simulink model "npc_controller"  (R2022a)
settings: Solver=FixedStepDiscrete  StartTime=0.0  StopTime=20  RelTol=1e-3  EnableMultiTasking=on
values from neighbouring files (symbols this model uses):
  Tsw = 1.5E-5    [param.sldd]
undefined symbols (not defined in the file or in its folder): CAN_O_INT, CANA_BASE, Down, GPTRIP1SEL, GPTRIP2SEL, GPTRIP3SEL, TZ1, TZ2, TZ3, Up
libraries: simulink x153, hdlsllib x90, c2802xlib x34, c2837xDlib x18, c280xlib x12, canmsglib x9, c2838xlib x8, idelinklib_common x3, c2806xlib x2, slpidlib x2, c28004xlib x2, c281xlib x2
(part 34 of 45)

== system npc_controller/CONTROL/CONTROL/false/CLA_CONTROL/CONTROL/vloop_pi_parallel ==
  note: okay til 0.1A load
  note: Parallel PI
  note: div10
  error : Inport
  Constant : Constant  Commented=on  Value=1.06066  OutDataTypeStr=single
  Constant1 : Constant  Commented=on  Value=0.00106066  OutDataTypeStr=single
  Constant10 : Constant  Commented=on  Value=0.000056066  OutDataTypeStr=single
  Constant11 : Constant  Value=-32*25.324  OutDataTypeStr=single
  Constant12 : Constant  Commented=on  Value=0  OutDataTypeStr=single
  Constant13 : Constant  Value=0.00056066  OutDataTypeStr=single
  Constant2 : Constant  Value=32*25.324  OutDataTypeStr=single
  Constant3 : Constant  Commented=on  Value=0.0056066  OutDataTypeStr=single
  Constant4 : Constant  OutDataTypeStr=single
  Constant5 : Constant  Value=0.56066  OutDataTypeStr=single
  Constant6 : Constant  Commented=on  Value=0.0056066  OutDataTypeStr=single
  Constant7 : Constant  Commented=on  Value=0.56066  OutDataTypeStr=single
  Constant8 : Constant  Commented=on  Value=0.00056066  OutDataTypeStr=single
  Constant9 : Constant  Commented=on  Value=0.056066  OutDataTypeStr=single
  Delay1 : Delay  DelayLength=1  InitialCondition=0  StateName=vbulk_pid1  StateMustResolveToSignalObject=on
  Product2 : Product  Inputs=3  OutDataTypeStr=single
  Product3 : Product  OutDataTypeStr=single
  Saturation Dynamic : simulink/Discontinuities/Saturation Dynamic  OutMin=[]  OutMax=[]  OutDataTypeStr=single  OutputDataTypeScalingMode=single  OutDataType=fixdt(1, 16)  OutScaling=2^-10  DoSatur=off
  Saturation Dynamic1 : simulink/Discontinuities/Saturation Dynamic  OutMin=[]  OutMax=[]  OutDataTypeStr=single  OutputDataTypeScalingMode=single  OutDataType=fixdt(1, 16)  OutScaling=2^-10  DoSatur=off
  Scope : Scope  NumInputPorts=4
  Sum : Sum  Inputs=|++  AccumDataTypeStr=single  OutDataTypeStr=single
  Sum3 : Sum  Inputs=|++  AccumDataTypeStr=single  OutDataTypeStr=single
  pi : Outport
  wires:
  [error] -> Scope/1  "error"
  [kP_term] -> Scope/2  "kP_term"
  [kI_term] -> Scope/3  "kI_term"
  [pi] -> Scope/4  "PI"
  [Ts] -> Product2/3
  Constant4/1 -> [Ts]
  [kp] -> Product3/2
  [integ_min] -> Saturation Dynamic/3
  Sum/1 -> Saturation Dynamic1/2
  [integ_min] -> Saturation Dynamic1/3
  [integ_max] -> Saturation Dynamic1/1
  Constant2/1 -> [integ_max]
  Constant11/1 -> [integ_min]
  Product2/1 -> Sum3/1
  Product3/1 -> Sum/1, [kP_term]
  [error] -> Product3/1
  Constant13/1 -> [ki]
  [integ_max] -> Saturation Dynamic/1
  [error] -> Product2/1
  error/1 -> [error]
  Saturation Dynamic/1 -> [kI_term], Sum/2, Delay1/1
  [ki] -> Product2/2
  Saturation Dynamic1/1 -> pi/1, [pi]
  Constant5/1 -> [kp]
  Sum3/1 -> Saturation Dynamic/2
  Delay1/1 -> Sum3/2

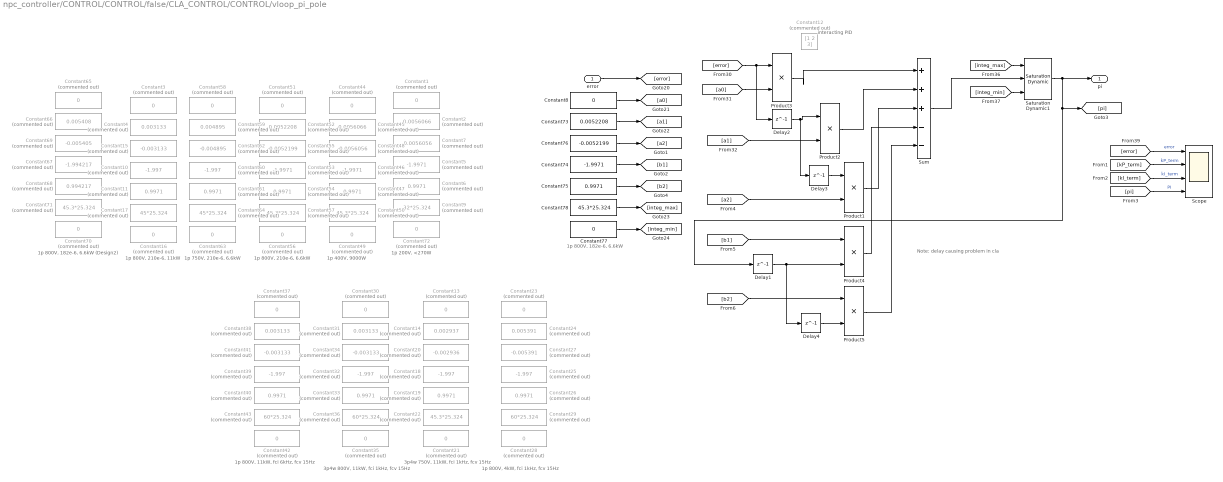
== system npc_controller/CONTROL/CONTROL/false/CLA_CONTROL/CONTROL/vloop_pi_pole ==
  note: interacting PID
  note: Note: delay causing problem in cla
  note: 1p 200V, <270W
  note: 3p4w 750V, 11kW, fci 1kHz, fcv 15Hz
  note: 1p 800V, 4kW, fci 1kHz, fcv 15Hz
  note: 3p4w 800V, 11kW, fci 1kHz, fcv 15Hz
  note: 1p 800V, 11kW, fci 6kHz, fcv 15Hz
  note: 1p 750V, 210e-6, 6.6kW
  note: 1p 800V, 210e-6, 6.6kW
  note: 1p 800V, 210e-6, 11kW
  note: 1p 800V, 182e-6, 6.6kW (Design2)
  note: 1p 400V, 9000W
  note: 1p 800V, 182e-6, 6.6kW
  error : Inport  OutDataTypeStr=single
  Constant{1,3,13,23,30,37,44,51,58,65} (10 alike) : Constant  Commented=on  Value=0  VectorParams1D=off  OutDataTypeStr=single
  Constant{10,18,25,32,39,60} (6 alike) : Constant  Commented=on  Value=-1.997  OutDataTypeStr=single
  Constant{6,11,19,26,33,40,47,54,61} (9 alike) : Constant  Commented=on  Value=0.9971  OutDataTypeStr=single
  Constant12 : Constant  Commented=on  Value=[1 2 3]  OutDataTypeStr=single
  Constant14 : Constant  Commented=on  Value=0.002937  OutDataTypeStr=single
  Constant15 : Constant  Commented=on  Value=-0.003133  OutDataTypeStr=single
  Constant{16,21,28,35,42,49,56,63,70,72} (10 alike) : Constant  Commented=on  Value=0  OutDataTypeStr=single
  Constant17 : Constant  Commented=on  Value=45*25.324  OutDataTypeStr=single
  Constant2 : Constant  Commented=on  Value=0.0056066  OutDataTypeStr=single
  Constant20 : Constant  Commented=on  Value=-0.002936  OutDataTypeStr=single
  Constant{22,50,57,71} (4 alike) : Constant  Commented=on  Value=45.3*25.324  OutDataTypeStr=single
  Constant24 : Constant  Commented=on  Value=0.005391  OutDataTypeStr=single
  Constant27 : Constant  Commented=on  Value=-0.005391  OutDataTypeStr=single
  Constant29 : Constant  Commented=on  Value=60*25.324  OutDataTypeStr=single
  Constant31 : Constant  Commented=on  Value=0.003133  OutDataTypeStr=single
  Constant34 : Constant  Commented=on  Value=-0.003133  OutDataTypeStr=single
  Constant36 : Constant  Commented=on  Value=60*25.324  OutDataTypeStr=single
  Constant38 : Constant  Commented=on  Value=0.003133  OutDataTypeStr=single
  Constant4 : Constant  Commented=on  Value=0.003133  OutDataTypeStr=single
  Constant41 : Constant  Commented=on  Value=-0.003133  OutDataTypeStr=single
  Constant43 : Constant  Commented=on  Value=60*25.324  OutDataTypeStr=single
  Constant45 : Constant  Commented=on  Value=0.0056066  OutDataTypeStr=single
  Constant46 : Constant  Commented=on  Value=-1.9971  OutDataTypeStr=single
  Constant48 : Constant  Commented=on  Value=-0.0056056  OutDataTypeStr=single
  Constant5 : Constant  Commented=on  Value=-1.9971  OutDataTypeStr=single
  Constant52 : Constant  Commented=on  Value=0.0052208  OutDataTypeStr=single
  Constant53 : Constant  Commented=on  Value=-1.9971  OutDataTypeStr=single
  Constant55 : Constant  Commented=on  Value=-0.0052199  OutDataTypeStr=single
  Constant59 : Constant  Commented=on  Value=0.004895  OutDataTypeStr=single
  Constant62 : Constant  Commented=on  Value=-0.004895  OutDataTypeStr=single
  Constant64 : Constant  Commented=on  Value=45*25.324  OutDataTypeStr=single
  Constant66 : Constant  Commented=on  Value=0.005408  OutDataTypeStr=single
  Constant67 : Constant  Commented=on  Value=-1.994217  OutDataTypeStr=single
  Constant68 : Constant  Commented=on  Value=0.994217  OutDataTypeStr=single
  Constant69 : Constant  Commented=on  Value=-0.005405  OutDataTypeStr=single
  Constant7 : Constant  Commented=on  Value=-0.0056056  OutDataTypeStr=single
  Constant73 : Constant  Value=0.0052208  OutDataTypeStr=single
  Constant74 : Constant  Value=-1.9971  OutDataTypeStr=single
  Constant75 : Constant  Value=0.9971  OutDataTypeStr=single
  Constant76 : Constant  Value=-0.0052199  OutDataTypeStr=single
  Constant77 : Constant  Value=0  OutDataTypeStr=single
  Constant78 : Constant  Value=45.3*25.324  OutDataTypeStr=single
  Constant8 : Constant  Value=0  VectorParams1D=off  OutDataTypeStr=single
  Constant9 : Constant  Commented=on  Value=32*25.324  OutDataTypeStr=single
  Delay1 : Delay  DelayLength=1  InitialCondition=0  StateName=vbulk_pid3  StateMustResolveToSignalObject=on
  Delay2 : Delay  DelayLength=1  InitialCondition=0  StateName=vbulk_pid1  StateMustResolveToSignalObject=on
  Delay3 : Delay  DelayLength=1  InitialCondition=0  StateName=vbulk_pid2  StateMustResolveToSignalObject=on
  Delay4 : Delay  DelayLength=1  InitialCondition=0  StateName=vbulk_pid4  StateMustResolveToSignalObject=on
  Product{1..5} (5 alike) : Product  OutDataTypeStr=single
  Saturation Dynamic1 : simulink/Discontinuities/Saturation Dynamic  OutMin=[]  OutMax=[]  OutDataTypeStr=single  OutputDataTypeScalingMode=single  OutDataType=fixdt(1, 16)  OutScaling=2^-10  DoSatur=off
  Scope : Scope  NumInputPorts=4
  Sum : Sum  Inputs=|+++--  AccumDataTypeStr=single  OutDataTypeStr=single
  pi : Outport
  wires:
  Constant75/1 -> [b2]
  Constant76/1 -> [a2]
  Constant74/1 -> [b1]
  [b2] -> Product5/1
  Product4/1 -> Sum/4
  Product5/1 -> Sum/5
  Delay4/1 -> Product5/2
  [b1] -> Product4/1
  Delay1/1 -> Delay4/1, Product4/2
  Product1/1 -> Sum/3
  Product2/1 -> Sum/2
  Product3/1 -> Sum/1
  [a2] -> Product1/2
  Delay3/1 -> Product1/1
  Saturation Dynamic1/1 -> [pi], Delay1/1, pi/1
  Delay2/1 -> Delay3/1, Product2/1
  [error] -> Product3/1, Delay2/1
  Constant8/1 -> [a0]
  [a1] -> Product2/2
  error/1 -> [error]
  Constant73/1 -> [a1]
  Constant77/1 -> [integ_min]
  Constant78/1 -> [integ_max]
  [integ_max] -> Saturation Dynamic1/1
  [integ_min] -> Saturation Dynamic1/3
  Sum/1 -> Saturation Dynamic1/2
  [a0] -> Product3/2
  [pi] -> Scope/4  "PI"
  [kI_term] -> Scope/3  "kI_term"
  [kP_term] -> Scope/2  "kP_term"
  [error] -> Scope/1  "error"

== system npc_controller/CONTROL/CONTROL/false/CLA_CONTROL/INIT//RESET_CONTROL/true ==
  Action Port : ActionPort  ActionPortLabel=if((u1 & u2 & u3) == 1)
  Constant{,1..13} (14 alike) : Constant  Commented=on  Value=0  OutDataTypeStr=single
  Constant{14..17} (4 alike) : Constant  Value=0  OutDataTypeStr=single
  State Writer : StateWriter  Commented=on
  State Writer1 : StateWriter  Commented=on
  State Writer10 : StateWriter  Commented=on  StateOwnerBlock=../../../CONTROL/pid_ic/Delay1  StateName=ic_pid3
  State Writer11 : StateWriter  Commented=on  StateOwnerBlock=../../../CONTROL/pid_ic/Delay2  StateName=ic_pid1
  State Writer12 : StateWriter  Commented=on  StateOwnerBlock=../../../CONTROL/pid_ic/Delay3  StateName=ic_pid2
  State Writer13 : StateWriter  Commented=on  StateOwnerBlock=../../../CONTROL/pid_ic/Delay4  StateName=ic_pid4
  State Writer14 : StateWriter  StateOwnerBlock=../../../CONTROL/vloop_pi_pole/Delay1  StateName=vbulk_pid3
  State Writer15 : StateWriter  StateOwnerBlock=../../../CONTROL/vloop_pi_pole/Delay2  StateName=vbulk_pid1
  State Writer16 : StateWriter  StateOwnerBlock=../../../CONTROL/vloop_pi_pole/Delay3  StateName=vbulk_pid2
  State Writer17 : StateWriter  StateOwnerBlock=../../../CONTROL/vloop_pi_pole/Delay4  StateName=vbulk_pid4
  State Writer2 : StateWriter  Commented=on  StateOwnerBlock=../../../CONTROL/pid_ia/Delay1  StateName=ia_pid3
  State Writer3 : StateWriter  Commented=on  StateOwnerBlock=../../../CONTROL/pid_ia/Delay2  StateName=ia_pid1
  State Writer4 : StateWriter  Commented=on  StateOwnerBlock=../../../CONTROL/pid_ia/Delay3  StateName=ia_pid2
  State Writer5 : StateWriter  Commented=on  StateOwnerBlock=../../../CONTROL/pid_ia/Delay4  StateName=ia_pid4
  State Writer6 : StateWriter  Commented=on  StateOwnerBlock=../../../CONTROL/pid_ib/Delay1  StateName=ib_pid3
  State Writer7 : StateWriter  Commented=on  StateOwnerBlock=../../../CONTROL/pid_ib/Delay2  StateName=ib_pid1
  State Writer8 : StateWriter  Commented=on  StateOwnerBlock=../../../CONTROL/pid_ib/Delay3  StateName=ib_pid2
  State Writer9 : StateWriter  Commented=on  StateOwnerBlock=../../../CONTROL/pid_ib/Delay4  StateName=ib_pid4
  wires:
  Constant/1 -> State Writer/1
  Constant1/1 -> State Writer1/1
  Constant2/1 -> State Writer2/1
  Constant3/1 -> State Writer3/1
  Constant4/1 -> State Writer4/1
  Constant5/1 -> State Writer5/1
  Constant6/1 -> State Writer6/1
  Constant7/1 -> State Writer7/1
  Constant8/1 -> State Writer8/1
  Constant9/1 -> State Writer9/1
  Constant10/1 -> State Writer10/1
  Constant11/1 -> State Writer11/1
  Constant12/1 -> State Writer12/1
  Constant13/1 -> State Writer13/1
  Constant17/1 -> State Writer17/1
  Constant16/1 -> State Writer16/1
  Constant14/1 -> State Writer14/1
  Constant15/1 -> State Writer15/1

== system npc_controller/CONTROL/CONTROL/false/CLA_CONTROL/INIT//RESET_CONTROL/true1 ==
  Action Port : ActionPort  ActionPortLabel=if(u1 == 0)
  Constant{,1,6..17} (14 alike) : Constant  Commented=on  Value=0  OutDataTypeStr=single
  Constant{2..5} (4 alike) : Constant  Value=0  OutDataTypeStr=single
  State Writer{,1,14..17} (6 alike) : StateWriter  Commented=on
  State Writer10 : StateWriter  Commented=on  StateOwnerBlock=../../../CONTROL/pid_ic/Delay1  StateName=ic_pid3
  State Writer11 : StateWriter  Commented=on  StateOwnerBlock=../../../CONTROL/pid_ic/Delay2  StateName=ic_pid1
  State Writer12 : StateWriter  Commented=on  StateOwnerBlock=../../../CONTROL/pid_ic/Delay3  StateName=ic_pid2
  State Writer13 : StateWriter  Commented=on  StateOwnerBlock=../../../CONTROL/pid_ic/Delay4  StateName=ic_pid4
  State Writer2 : StateWriter  StateOwnerBlock=../../../CONTROL/pid_ia/Delay1  StateName=ia_pid3
  State Writer3 : StateWriter  StateOwnerBlock=../../../CONTROL/pid_ia/Delay2  StateName=ia_pid1
  State Writer4 : StateWriter  StateOwnerBlock=../../../CONTROL/pid_ia/Delay3  StateName=ia_pid2
  State Writer5 : StateWriter  StateOwnerBlock=../../../CONTROL/pid_ia/Delay4  StateName=ia_pid4
  State Writer6 : StateWriter  Commented=on  StateOwnerBlock=../../../CONTROL/pid_ib/Delay1  StateName=ib_pid3
  State Writer7 : StateWriter  Commented=on  StateOwnerBlock=../../../CONTROL/pid_ib/Delay2  StateName=ib_pid1
  State Writer8 : StateWriter  Commented=on  StateOwnerBlock=../../../CONTROL/pid_ib/Delay3  StateName=ib_pid2
  State Writer9 : StateWriter  Commented=on  StateOwnerBlock=../../../CONTROL/pid_ib/Delay4  StateName=ib_pid4
  wires:
  Constant15/1 -> State Writer15/1
  Constant14/1 -> State Writer14/1
  Constant16/1 -> State Writer16/1
  Constant17/1 -> State Writer17/1
  Constant13/1 -> State Writer13/1
  Constant12/1 -> State Writer12/1
  Constant11/1 -> State Writer11/1
  Constant10/1 -> State Writer10/1
  Constant9/1 -> State Writer9/1
  Constant8/1 -> State Writer8/1
  Constant7/1 -> State Writer7/1
  Constant6/1 -> State Writer6/1
  Constant5/1 -> State Writer5/1
  Constant4/1 -> State Writer4/1
  Constant3/1 -> State Writer3/1
  Constant2/1 -> State Writer2/1
  Constant1/1 -> State Writer1/1
  Constant/1 -> State Writer/1

== system npc_controller/CONTROL/CONTROL/false/CLA_CONTROL/INIT//RESET_CONTROL/true2 ==
  Action Port : ActionPort  ActionPortLabel=if(u1 == 0)
  Constant{,1..5,10..17} (14 alike) : Constant  Commented=on  Value=0  OutDataTypeStr=single
  Constant{6..9} (4 alike) : Constant  Value=0  OutDataTypeStr=single
  State Writer{,1,14..17} (6 alike) : StateWriter  Commented=on
  State Writer10 : StateWriter  Commented=on  StateOwnerBlock=../../../CONTROL/pid_ic/Delay1  StateName=ic_pid3
  State Writer11 : StateWriter  Commented=on  StateOwnerBlock=../../../CONTROL/pid_ic/Delay2  StateName=ic_pid1
  State Writer12 : StateWriter  Commented=on  StateOwnerBlock=../../../CONTROL/pid_ic/Delay3  StateName=ic_pid2
  State Writer13 : StateWriter  Commented=on  StateOwnerBlock=../../../CONTROL/pid_ic/Delay4  StateName=ic_pid4
  State Writer2 : StateWriter  Commented=on  StateOwnerBlock=../../../CONTROL/pid_ia/Delay1  StateName=ia_pid3
  State Writer3 : StateWriter  Commented=on  StateOwnerBlock=../../../CONTROL/pid_ia/Delay2  StateName=ia_pid1
  State Writer4 : StateWriter  Commented=on  StateOwnerBlock=../../../CONTROL/pid_ia/Delay3  StateName=ia_pid2
  State Writer5 : StateWriter  Commented=on  StateOwnerBlock=../../../CONTROL/pid_ia/Delay4  StateName=ia_pid4
  State Writer6 : StateWriter  StateOwnerBlock=../../../CONTROL/pid_ib/Delay1  StateName=ib_pid3
  State Writer7 : StateWriter  StateOwnerBlock=../../../CONTROL/pid_ib/Delay2  StateName=ib_pid1
  State Writer8 : StateWriter  StateOwnerBlock=../../../CONTROL/pid_ib/Delay3  StateName=ib_pid2
  State Writer9 : StateWriter  StateOwnerBlock=../../../CONTROL/pid_ib/Delay4  StateName=ib_pid4
  wires:
  Constant/1 -> State Writer/1
  Constant1/1 -> State Writer1/1
  Constant2/1 -> State Writer2/1
  Constant3/1 -> State Writer3/1
  Constant4/1 -> State Writer4/1
  Constant5/1 -> State Writer5/1
  Constant6/1 -> State Writer6/1
  Constant7/1 -> State Writer7/1
  Constant8/1 -> State Writer8/1
  Constant9/1 -> State Writer9/1
  Constant10/1 -> State Writer10/1
  Constant11/1 -> State Writer11/1
  Constant12/1 -> State Writer12/1
  Constant13/1 -> State Writer13/1
  Constant17/1 -> State Writer17/1
  Constant16/1 -> State Writer16/1
  Constant14/1 -> State Writer14/1
  Constant15/1 -> State Writer15/1

== system npc_controller/CONTROL/CONTROL/false/CLA_CONTROL/INIT//RESET_CONTROL/true3 ==
  Action Port : ActionPort  ActionPortLabel=if(u1 == 0)
  Constant{,1..9,14..17} (14 alike) : Constant  Commented=on  Value=0  OutDataTypeStr=single
  Constant{10..13} (4 alike) : Constant  Value=0  OutDataTypeStr=single
  State Writer{,1,14..17} (6 alike) : StateWriter  Commented=on
  State Writer10 : StateWriter  StateOwnerBlock=../../../CONTROL/pid_ic/Delay1  StateName=ic_pid3
  State Writer11 : StateWriter  StateOwnerBlock=../../../CONTROL/pid_ic/Delay2  StateName=ic_pid1
  State Writer12 : StateWriter  StateOwnerBlock=../../../CONTROL/pid_ic/Delay3  StateName=ic_pid2
  State Writer13 : StateWriter  StateOwnerBlock=../../../CONTROL/pid_ic/Delay4  StateName=ic_pid4
  State Writer2 : StateWriter  Commented=on  StateOwnerBlock=../../../CONTROL/pid_ia/Delay1  StateName=ia_pid3
  State Writer3 : StateWriter  Commented=on  StateOwnerBlock=../../../CONTROL/pid_ia/Delay2  StateName=ia_pid1
  State Writer4 : StateWriter  Commented=on  StateOwnerBlock=../../../CONTROL/pid_ia/Delay3  StateName=ia_pid2
  State Writer5 : StateWriter  Commented=on  StateOwnerBlock=../../../CONTROL/pid_ia/Delay4  StateName=ia_pid4
  State Writer6 : StateWriter  Commented=on  StateOwnerBlock=../../../CONTROL/pid_ib/Delay1  StateName=ib_pid3
  State Writer7 : StateWriter  Commented=on  StateOwnerBlock=../../../CONTROL/pid_ib/Delay2  StateName=ib_pid1
  State Writer8 : StateWriter  Commented=on  StateOwnerBlock=../../../CONTROL/pid_ib/Delay3  StateName=ib_pid2
  State Writer9 : StateWriter  Commented=on  StateOwnerBlock=../../../CONTROL/pid_ib/Delay4  StateName=ib_pid4
  wires:
  Constant15/1 -> State Writer15/1
  Constant14/1 -> State Writer14/1
  Constant16/1 -> State Writer16/1
  Constant17/1 -> State Writer17/1
  Constant13/1 -> State Writer13/1
  Constant12/1 -> State Writer12/1
  Constant11/1 -> State Writer11/1
  Constant10/1 -> State Writer10/1
  Constant9/1 -> State Writer9/1
  Constant8/1 -> State Writer8/1
  Constant7/1 -> State Writer7/1
  Constant6/1 -> State Writer6/1
  Constant5/1 -> State Writer5/1
  Constant4/1 -> State Writer4/1
  Constant3/1 -> State Writer3/1
  Constant2/1 -> State Writer2/1
  Constant1/1 -> State Writer1/1
  Constant/1 -> State Writer/1

== system npc_controller/CONTROL/GET_ADC/ADC/codegen/ADCA/Subsystem10 ==
  In1 : Inport
  Cast To Single1 : DataTypeConversion  Commented=on  OutDataTypeStr=uint16  SaturateOnIntegerOverflow=off  RndMeth=Floor
  Data Store Read4 : DataStoreRead  DataStoreName=adc_offset_vb  IndexOptions=Index vector (dialog)  Indices=1  OutputSizes=1
  Data Store Write3 : DataStoreWrite  DataStoreName=adc_vb  IndexOptions=Index vector (dialog)  Indices=1  OutputSizes=1
  vabc3 : Sum  Inputs=|+-  AccumDataTypeStr=single  OutDataTypeStr=single
  Outport : Outport
  wires:
  Data Store Read4/1 -> vabc3/2
  vabc3/1 -> Outport/1
  In1/1 -> Cast To Single1/1, Data Store Write3/1, vabc3/1  "va"

== system npc_controller/CONTROL/GET_ADC/ADC/codegen/ADCA/Subsystem11 ==
  x[n] : Inport
  Cast To Single1 : DataTypeConversion  Commented=on  OutDataTypeStr=uint16  SaturateOnIntegerOverflow=off  RndMeth=Floor
  Cast To Single4 : DataTypeConversion  OutDataTypeStr=uint16  SaturateOnIntegerOverflow=off  RndMeth=Floor
  Data Store Read4 : DataStoreRead  DataStoreName=adc_offset_vc  IndexOptions=Index vector (dialog)  Indices=1  OutputSizes=1
  Data Store Write2 : DataStoreWrite  DataStoreName=u16Debug2  IndexOptions=Index vector (dialog)  Indices=1  OutputSizes=1
  Data Store Write3 : DataStoreWrite  DataStoreName=adc_vc  IndexOptions=Index vector (dialog)  Indices=1  OutputSizes=1
  vabc3 : Sum  Inputs=|+-  AccumDataTypeStr=single  OutDataTypeStr=single
  Outport : Outport
  wires:
  Data Store Read4/1 -> Cast To Single4/1, vabc3/2
  x[n]/1 -> Cast To Single1/1, Data Store Write3/1, vabc3/1  "va"
  vabc3/1 -> Outport/1
  Cast To Single4/1 -> Data Store Write2/1
  Cast To Single1/1 -> ?

== system npc_controller/CONTROL/GET_ADC/ADC/codegen/ADCA/Subsystem17 ==
  Inport : Inport
  Data Store Write : DataStoreWrite  DataStoreName=adc_temp_mux  IndexOptions=Index vector (dialog)  Indices=1  OutputSizes=1
  wires:
  Inport/1 -> Data Store Write/1

== system npc_controller/CONTROL/GET_ADC/ADC/codegen/ADCA/Subsystem18 ==
  In1 : Inport
  Data Store Write12 : DataStoreWrite  DataStoreName=adc_vaux  IndexOptions=Index vector (dialog)  Indices=1  OutputSizes=1
  wires:
  In1/1 -> Data Store Write12/1

== system npc_controller/CONTROL/GET_ADC/ADC/codegen/ADCA/Subsystem6 ==
  note: +-30Apeak
  note: //3040 = 40A , 1055 = -40A
  note: +-20Apeak
  Input : Inport
  Data Store Read4 : DataStoreRead  DataStoreName=adc_offset_ic  IndexOptions=Index vector (dialog)  Indices=1  OutputSizes=1
  Data Store Read6 : DataStoreRead  DataStoreName=ac_ok  IndexOptions=Index vector (dialog)  Indices=1  OutputSizes=1
  Data Store Write3 : DataStoreWrite  DataStoreName=adc_ic  IndexOptions=Index vector (dialog)  Indices=1  OutputSizes=1
  If : If  Commented=on  IfExpression=(u1 > 2979) | (u1 < 1525)
  If Action Subsystem : Subsystem  Commented=on  TreatAsAtomicUnit=on
  If Action Subsystem1 : Subsystem  TreatAsAtomicUnit=on
  If Action Subsystem2 : Subsystem  TreatAsAtomicUnit=on
  If1 : If  Commented=on  IfExpression=(u1 > 3040) | (u1 < 1055)
  If2 : If  Commented=on  IfExpression=(u1 > 2736) | (u1 < 1767)
  If3 : If  IfExpression=u1 == 0
  calib : Subsystem  Commented=on
  vabc3 : Sum  Inputs=|+-  AccumDataTypeStr=single  OutDataTypeStr=single
  Outport : Outport
  wires:
  Data Store Read4/1 -> vabc3/2
  vabc3/1 -> Outport/1
  If/1 -> If Action Subsystem/Action
  Data Store Read6/1 -> If3/1
  If3/2 -> If Action Subsystem1/Action
  Input/1 -> If Action Subsystem2/1(Input), If Action Subsystem1/1(Input), Data Store Write3/1, vabc3/1
  If3/1 -> If Action Subsystem2/Action

== system npc_controller/CONTROL/GET_ADC/ADC/codegen/ADCA/Subsystem7 ==
  note: //3040 = 40A , 1055 = -40A
  note: +-20Apeak
  note: +-30Apeak
  note: //3221 = 40A , 1283 = -40A
  x[n] : Inport
  Data Store Read4 : DataStoreRead  DataStoreName=adc_offset_ib  IndexOptions=Index vector (dialog)  Indices=1  OutputSizes=1
  Data Store Read6 : DataStoreRead  DataStoreName=ac_ok  IndexOptions=Index vector (dialog)  Indices=1  OutputSizes=1
  Data Store Write3 : DataStoreWrite  DataStoreName=adc_ib  IndexOptions=Index vector (dialog)  Indices=1  OutputSizes=1
  If : If  Commented=on  IfExpression=(u1 > 3040) | (u1 < 1055)
  If Action Subsystem : Subsystem  Commented=on  TreatAsAtomicUnit=on
  If Action Subsystem1 : Subsystem  TreatAsAtomicUnit=on
  If Action Subsystem2 : Subsystem  TreatAsAtomicUnit=on
  If1 : If  Commented=on  IfExpression=(u1 > 2736) | (u1 < 1767)
  If2 : If  Commented=on  IfExpression=(u1 > 2979) | (u1 < 1525)
  If3 : If  IfExpression=u1 == 0
  If4 : If  Commented=on  IfExpression=(u1 > 3221) | (u1 < 1283)
  calib : Subsystem  Commented=on
  vabc3 : Sum  Inputs=|+-  AccumDataTypeStr=single  OutDataTypeStr=single
  Outport : Outport
  wires:
  Data Store Read4/1 -> vabc3/2
  vabc3/1 -> Outport/1
  If2/1 -> If Action Subsystem/Action
  If3/1 -> If Action Subsystem2/Action
  If3/2 -> If Action Subsystem1/Action
  x[n]/1 -> If Action Subsystem2/1(Input), If Action Subsystem1/1(Input), Data Store Write3/1, vabc3/1
  Data Store Read6/1 -> If3/1

== system npc_controller/CONTROL/GET_ADC/ADC/codegen/ADCA/Subsystem8 ==
  note: +40, -40A
  note: //3040 = 40A , 1055 = -40A
      | //2544 = 20A , 1553 = -20A
  note: +-20Apeak
  Input : Inport
  Data Store Read4 : DataStoreRead  DataStoreName=adc_offset_ia  IndexOptions=Index vector (dialog)  Indices=1  OutputSizes=1
  Data Store Read6 : DataStoreRead  DataStoreName=ac_ok  IndexOptions=Index vector (dialog)  Indices=1  OutputSizes=1
  Data Store Write3 : DataStoreWrite  DataStoreName=adc_ia  IndexOptions=Index vector (dialog)  Indices=1  OutputSizes=1
  If : If  Commented=on  IfExpression=(u1 > 3040) | (u1 < 1055)
  If Action Subsystem1 : Subsystem  TreatAsAtomicUnit=on
  If Action Subsystem2 : Subsystem  TreatAsAtomicUnit=on
  If2 : If  Commented=on  IfExpression=(u1 > 2736) | (u1 < 1767)
  If3 : If  IfExpression=u1 == 0
  calib : Subsystem  Commented=on
  vabc3 : Sum  Inputs=|+-  AccumDataTypeStr=single  OutDataTypeStr=single
  Outport : Outport
  wires:
  Data Store Read4/1 -> vabc3/2
  vabc3/1 -> Outport/1
  Input/1 -> If Action Subsystem2/1(Input), If Action Subsystem1/1(Input), Data Store Write3/1, vabc3/1
  If3/2 -> If Action Subsystem1/Action
  If3/1 -> If Action Subsystem2/Action
  Data Store Read6/1 -> If3/1

== system npc_controller/CONTROL/GET_ADC/ADC/codegen/ADCA/Subsystem9 ==
  x[n] : Inport
  Cast To Single4 : DataTypeConversion  OutDataTypeStr=uint16  SaturateOnIntegerOverflow=off  RndMeth=Floor
  Data Store Read4 : DataStoreRead  DataStoreName=adc_offset_va  IndexOptions=Index vector (dialog)  Indices=1  OutputSizes=1
  Data Store Write2 : DataStoreWrite  DataStoreName=u16Debug3  IndexOptions=Index vector (dialog)  Indices=1  OutputSizes=1
  Data Store Write3 : DataStoreWrite  DataStoreName=adc_va  IndexOptions=Index vector (dialog)  Indices=1  OutputSizes=1
  vabc3 : Sum  Inputs=|+-  AccumDataTypeStr=single  OutDataTypeStr=single
  Outport : Outport
  wires:
  Data Store Read4/1 -> vabc3/2
  vabc3/1 -> Outport/1
  x[n]/1 -> Cast To Single4/1, Data Store Write3/1, vabc3/1
  Cast To Single4/1 -> Data Store Write2/1

== system npc_controller/CONTROL/GET_ADC/ADC/codegen/ADCC/Subsystem12 ==
  In1 : Inport
  Data Store Write8 : DataStoreWrite  DataStoreName=adc_vmid  IndexOptions=Index vector (dialog)  Indices=1  OutputSizes=1
  Outport : Outport
  wires:
  In1/1 -> Data Store Write8/1, Outport/1

== system npc_controller/CONTROL/GET_ADC/ADC/codegen/ADCC/Subsystem13 ==
  x[n] : Inport
  Data Store Write6 : DataStoreWrite  DataStoreName=adc_vbulk  IndexOptions=Index vector (dialog)  Indices=1  OutputSizes=1
  Outport : Outport
  wires:
  x[n]/1 -> Outport/1, Data Store Write6/1

== system npc_controller/CONTROL/GET_ADC/ADC/codegen/ADCC/Subsystem14 ==
  In1 : Inport
  Data Store Read4 : DataStoreRead  DataStoreName=adc_offset_ia  IndexOptions=Index vector (dialog)  Indices=1  OutputSizes=1
  Data Store Write46 : DataStoreWrite  DataStoreName=adc_iphasea  IndexOptions=Index vector (dialog)  Indices=1  OutputSizes=1
  vabc3 : Sum  Inputs=|+-  AccumDataTypeStr=single  OutDataTypeStr=single
  iphasea : Outport
  wires:
  vabc3/1 -> Data Store Write46/1, iphasea/1
  Data Store Read4/1 -> vabc3/2
  In1/1 -> vabc3/1

== system npc_controller/CONTROL/GET_ADC/ADC/codegen/ADCC/Subsystem15 ==
  In1 : Inport
  Data Store Read4 : DataStoreRead  DataStoreName=adc_offset_ib  IndexOptions=Index vector (dialog)  Indices=1  OutputSizes=1
  Data Store Write46 : DataStoreWrite  DataStoreName=adc_iphaseb  IndexOptions=Index vector (dialog)  Indices=1  OutputSizes=1
  vabc3 : Sum  Inputs=|+-  AccumDataTypeStr=single  OutDataTypeStr=single
  iphaseb : Outport
  wires:
  vabc3/1 -> Data Store Write46/1, iphaseb/1
  Data Store Read4/1 -> vabc3/2
  In1/1 -> vabc3/1

== system npc_controller/CONTROL/GET_ADC/ADC/codegen/ADCC/Subsystem16 ==
  In1 : Inport
  Data Store Read4 : DataStoreRead  DataStoreName=adc_offset_ic  IndexOptions=Index vector (dialog)  Indices=1  OutputSizes=1
  Data Store Write46 : DataStoreWrite  DataStoreName=adc_iphasec  IndexOptions=Index vector (dialog)  Indices=1  OutputSizes=1
  vabc3 : Sum  Inputs=|+-  AccumDataTypeStr=single  OutDataTypeStr=single
  iphasec : Outport
  wires:
  vabc3/1 -> Data Store Write46/1, iphasec/1
  Data Store Read4/1 -> vabc3/2
  In1/1 -> vabc3/1

== system npc_controller/CONTROL/GET_ADC/ADC/codegen/Subsystem/IIR Filter1 ==
  note: 10 half cycles of 50Hz
      |
      | 1/(5*650)
  note: prev 0.98
  x[n] : Inport
  1 - Lambda : Gain  Gain=0.00015384  ParamDataTypeStr=single  OutDataTypeStr=single
  Delay : Delay  DelayLength=1
  Lambda : Gain  Gain=0.99984615  ParamDataTypeStr=single  OutDataTypeStr=single
  Sum : Sum  Inputs=|++  AccumDataTypeStr=single  OutDataTypeStr=single
  y[n] : Outport
  wires:
  Delay/1 -> Lambda/1
  Lambda/1 -> Sum/2
  Sum/1 -> y[n]/1, Delay/1
  1 - Lambda/1 -> Sum/1
  x[n]/1 -> 1 - Lambda/1

== system npc_controller/CONTROL/GET_ADC/ADC/codegen/Subsystem1/IIR Filter1 ==
  note: 10 half cycles of 50Hz
      |
      | 1/(5*650)
  note: prev 0.98
  x[n] : Inport
  1 - Lambda : Gain  Gain=0.00015384  ParamDataTypeStr=single  OutDataTypeStr=single
  Delay : Delay  DelayLength=1
  Lambda : Gain  Gain=0.99984615  ParamDataTypeStr=single  OutDataTypeStr=single
  Sum : Sum  Inputs=|++  AccumDataTypeStr=single  OutDataTypeStr=single
  y[n] : Outport
  wires:
  Delay/1 -> Lambda/1
  Lambda/1 -> Sum/2
  Sum/1 -> y[n]/1, Delay/1
  1 - Lambda/1 -> Sum/1
  x[n]/1 -> 1 - Lambda/1

== system npc_controller/CONTROL/GET_ADC/ADC/codegen/Subsystem2/IIR Filter1 ==
  note: 10 half cycles of 50Hz
      |
      | 1/(5*650)
  note: prev 0.98
  x[n] : Inport
  1 - Lambda : Gain  Gain=0.00015384  ParamDataTypeStr=single  OutDataTypeStr=single
  Delay : Delay  DelayLength=1
  Lambda : Gain  Gain=0.99984615  ParamDataTypeStr=single  OutDataTypeStr=single
  Sum : Sum  Inputs=|++  AccumDataTypeStr=single  OutDataTypeStr=single
  y[n] : Outport
  wires:
  Delay/1 -> Lambda/1
  Lambda/1 -> Sum/2
  Sum/1 -> y[n]/1, Delay/1
  1 - Lambda/1 -> Sum/1
  x[n]/1 -> 1 - Lambda/1

== system npc_controller/CONTROL/GET_ADC/ADC/codegen/Subsystem3/IIR Filter1 ==
  note: 10 half cycles of 50Hz
      |
      | 1/(5*650)
  note: prev 0.98
  x[n] : Inport
  1 - Lambda : Gain  Gain=0.00015384  ParamDataTypeStr=single  OutDataTypeStr=single
  Delay : Delay  DelayLength=1
  Lambda : Gain  Gain=0.99984615  ParamDataTypeStr=single  OutDataTypeStr=single
  Sum : Sum  Inputs=|++  AccumDataTypeStr=single  OutDataTypeStr=single
  y[n] : Outport
  wires:
  Delay/1 -> Lambda/1
  Lambda/1 -> Sum/2
  Sum/1 -> y[n]/1, Delay/1
  1 - Lambda/1 -> Sum/1
  x[n]/1 -> 1 - Lambda/1

== system npc_controller/CONTROL/GET_ADC/ADC/codegen/Subsystem4/IIR Filter1 ==
  note: 10 half cycles of 50Hz
      |
      | 1/(5*650)
  note: prev 0.98
  x[n] : Inport
  1 - Lambda : Gain  Gain=0.00015384  ParamDataTypeStr=single  OutDataTypeStr=single
  Delay : Delay  DelayLength=1
  Lambda : Gain  Gain=0.99984615  ParamDataTypeStr=single  OutDataTypeStr=single
  Sum : Sum  Inputs=|++  AccumDataTypeStr=single  OutDataTypeStr=single
  y[n] : Outport
  wires:
  Delay/1 -> Lambda/1
  Lambda/1 -> Sum/2
  Sum/1 -> y[n]/1, Delay/1
  1 - Lambda/1 -> Sum/1
  x[n]/1 -> 1 - Lambda/1

== system npc_controller/CONTROL/GET_ADC/ADC/codegen/Subsystem5/IIR Filter1 ==
  note: 10 half cycles of 50Hz
      |
      | 1/(5*650)
  note: prev 0.98
  x[n] : Inport
  1 - Lambda : Gain  Gain=0.00015384  ParamDataTypeStr=single  OutDataTypeStr=single
  Delay : Delay  DelayLength=1
  Lambda : Gain  Gain=0.99984615  ParamDataTypeStr=single  OutDataTypeStr=single
  Sum : Sum  Inputs=|++  AccumDataTypeStr=single  OutDataTypeStr=single
  y[n] : Outport
  wires:
  Delay/1 -> Lambda/1
  Lambda/1 -> Sum/2
  Sum/1 -> y[n]/1, Delay/1
  1 - Lambda/1 -> Sum/1
  x[n]/1 -> 1 - Lambda/1

== system npc_controller/CONTROL/GET_ADC/ADC/codegen/Subsystem6/IIR Filter1 ==
  note: prev 0.98
  note: 10 half cycles of 50Hz
      |
      | 1/(5*650)
  x[n] : Inport
  1 - Lambda : Gain  Gain=0.00015384  ParamDataTypeStr=single  OutDataTypeStr=single
  Delay : Delay  DelayLength=1
  Lambda : Gain  Gain=0.99984615  ParamDataTypeStr=single  OutDataTypeStr=single
  Sum : Sum  Inputs=|++  AccumDataTypeStr=single  OutDataTypeStr=single
  y[n] : Outport
  wires:
  x[n]/1 -> 1 - Lambda/1
  1 - Lambda/1 -> Sum/1
  Sum/1 -> Delay/1, y[n]/1
  Lambda/1 -> Sum/2
  Delay/1 -> Lambda/1

== system npc_controller/CONTROL/GET_ADC/ADC/codegen/Subsystem7/IIR Filter1 ==
  note: prev 0.98
  note: 10 half cycles of 50Hz
      |
      | 1/(5*650)
  x[n] : Inport
  1 - Lambda : Gain  Gain=0.00015384  ParamDataTypeStr=single  OutDataTypeStr=single
  Delay : Delay  DelayLength=1
  Lambda : Gain  Gain=0.99984615  ParamDataTypeStr=single  OutDataTypeStr=single
  Sum : Sum  Inputs=|++  AccumDataTypeStr=single  OutDataTypeStr=single
  y[n] : Outport
  wires:
  x[n]/1 -> 1 - Lambda/1
  1 - Lambda/1 -> Sum/1
  Sum/1 -> Delay/1, y[n]/1
  Lambda/1 -> Sum/2
  Delay/1 -> Lambda/1

== system npc_controller/CONTROL/GET_ADC/ADC/codegen/Subsystem8/IIR Filter1 ==
  note: prev 0.98
  note: 10 half cycles of 50Hz
      |
      | 1/(5*650)
  x[n] : Inport
  1 - Lambda : Gain  Gain=0.00015384  ParamDataTypeStr=single  OutDataTypeStr=single
  Delay : Delay  DelayLength=1
  Lambda : Gain  Gain=0.99984615  ParamDataTypeStr=single  OutDataTypeStr=single
  Sum : Sum  Inputs=|++  AccumDataTypeStr=single  OutDataTypeStr=single
  y[n] : Outport
  wires:
  x[n]/1 -> 1 - Lambda/1
  1 - Lambda/1 -> Sum/1
  Sum/1 -> Delay/1, y[n]/1
  Lambda/1 -> Sum/2
  Delay/1 -> Lambda/1

== system npc_controller/CONTROL/POLARITY/PLL_Block1/SRF_PLL/Integrator/Accumulation ==
  In1 : Inport  OutDataTypeStr=single
  Action Port : ActionPort
  Out : Outport  OutDataTypeStr=single
  wires:
  In1/1 -> Out/1

== system npc_controller/CONTROL/POLARITY/PLL_Block1/SRF_PLL/Integrator/Reset Integrator ==
  Action Port : ActionPort
  Constant1 : Constant  Value=0  OutDataTypeStr=single
  Out : Outport
  wires:
  Constant1/1 -> Out/1

== system npc_controller/CONTROL/STATE-MACHINE/CPU_CONTROL_100_A2_precharge_pfc_ok2/configGrid/FORCE_TZ/1P/ALL_LEGS ==
  note: Note:
      | TZCCTL
      | 0b00 - High impedance
      | 0b01 - Force to HIGH
      | 0b10 - Force to LOW
      | 0b11 - Do nothing
      |
      | AQCSFRC
      | 0b00 - disables forced PWM
      | 0b01 - forces PWM to LOW
      | 0b10 - forces PWM to  HIGH
      |
      | TZFRC.bit.OST
      | 0b0 - Do nothing
      | 0b1 - Force TZ
  note: EALLOW;
      |
      | /*Force TZ*/
      | EPwm6Regs. TZFRC.bit.OST = 0b0; //do nothing
      | EPwm7Regs. TZFRC.bit.OST = 0b0;
      | EPwm8Regs. TZFRC.bit.OST = 0b0;
      | EPwm9Regs. TZFRC.bit.OST = 0b0;
      | EPwm10Regs. TZFRC.bit.OST = 0b0;
      | EPwm11Regs. TZFRC.bit.OST = 0b0;
      |
      | EDIS;
      |
      | //change ref for leg B and legC
  Action Port : ActionPort
  System Outputs2 : Subsystem  mask(System Outputs){ShowInLibBrowser=0}
      mask prompts: ShowInLibBrowser "Simulink:masks:CustCodeMaskParam1_MP"
      settings: CopyFcn=cccopyfcn(gcb)  OpenFcn=ccopenfcn('System Outputs Function')
      mask Help: eval('feval(''rtwprivate'',''rtwhelpview'',''rtw_sys_outputs_block'')');
      mask Display: disp('System\nOutputs');

== system npc_controller/CONTROL/STATE-MACHINE/CPU_CONTROL_100_A2_precharge_pfc_ok2/configGrid/FORCE_TZ/1P/LEG_A ==
  note: EALLOW;
      |
      | /*Force TZ*/
      | EPwm6Regs. TZFRC.bit.OST = 0b0; //do nothing
      | EPwm7Regs. TZFRC.bit.OST = 0b0;
      | EPwm8Regs. TZFRC.bit.OST = 0b1;
      | EPwm9Regs. TZFRC.bit.OST = 0b1;
      | EPwm10Regs. TZFRC.bit.OST = 0b1;
      | EPwm11Regs. TZFRC.bit.OST = 0b1;
      |
      | EDIS;
  note: Note:
      | TZCCTL
      | 0b00 - High impedance
      | 0b01 - Force to HIGH
      | 0b10 - Force to LOW
      | 0b11 - Do nothing
      |
      | AQCSFRC
      | 0b00 - disables forced PWM
      | 0b01 - forces PWM to LOW
      | 0b10 - forces PWM to  HIGH
      |
      | TZFRC.bit.OST
      | 0b0 - Do nothing
      | 0b1 - Force TZ
  Action Port : ActionPort
  System Outputs2 : Subsystem  mask(System Outputs){ShowInLibBrowser=0}
      mask prompts: ShowInLibBrowser "Simulink:masks:CustCodeMaskParam1_MP"
      settings: CopyFcn=cccopyfcn(gcb)  OpenFcn=ccopenfcn('System Outputs Function')
      mask Help: eval('feval(''rtwprivate'',''rtwhelpview'',''rtw_sys_outputs_block'')');
      mask Display: disp('System\nOutputs');

== system npc_controller/CONTROL/STATE-MACHINE/CPU_CONTROL_100_A2_precharge_pfc_ok2/configGrid/FORCE_TZ/1P/LEG_B ==
  note: Note:
      | TZCCTL
      | 0b00 - High impedance
      | 0b01 - Force to HIGH
      | 0b10 - Force to LOW
      | 0b11 - Do nothing
      |
      | AQCSFRC
      | 0b00 - disables forced PWM
      | 0b01 - forces PWM to LOW
      | 0b10 - forces PWM to  HIGH
      |
      | TZFRC.bit.OST
      | 0b0 - Do nothing
      | 0b1 - Force TZ
  note: EALLOW;
      |
      | /*Force TZ*/
      | EPwm6Regs. TZFRC.bit.OST = 0b1; //do nothing
      | EPwm7Regs. TZFRC.bit.OST = 0b1;
      | EPwm8Regs. TZFRC.bit.OST = 0b0;
      | EPwm9Regs. TZFRC.bit.OST = 0b0;
      | EPwm10Regs. TZFRC.bit.OST = 0b1;
      | EPwm11Regs. TZFRC.bit.OST = 0b1;
      |
      | EDIS;
  Action Port : ActionPort
  System Outputs2 : Subsystem  mask(System Outputs){ShowInLibBrowser=0}
      mask prompts: ShowInLibBrowser "Simulink:masks:CustCodeMaskParam1_MP"
      settings: CopyFcn=cccopyfcn(gcb)  OpenFcn=ccopenfcn('System Outputs Function')
      mask Help: eval('feval(''rtwprivate'',''rtwhelpview'',''rtw_sys_outputs_block'')');
      mask Display: disp('System\nOutputs');

== system npc_controller/CONTROL/STATE-MACHINE/CPU_CONTROL_100_A2_precharge_pfc_ok2/configGrid/FORCE_TZ/1P/LEG_C ==
  note: EALLOW;
      |
      | /*Force TZ*/
      | EPwm6Regs. TZFRC.bit.OST = 0b1; //do nothing
      | EPwm7Regs. TZFRC.bit.OST = 0b1;
      | EPwm8Regs. TZFRC.bit.OST = 0b1;
      | EPwm9Regs. TZFRC.bit.OST = 0b1;
      | EPwm10Regs. TZFRC.bit.OST = 0b0;
      | EPwm11Regs. TZFRC.bit.OST = 0b0;
      |
      | EDIS;
  note: Note:
      | TZCCTL
      | 0b00 - High impedance
      | 0b01 - Force to HIGH
      | 0b10 - Force to LOW
      | 0b11 - Do nothing
      |
      | AQCSFRC
      | 0b00 - disables forced PWM
      | 0b01 - forces PWM to LOW
      | 0b10 - forces PWM to  HIGH
      |
      | TZFRC.bit.OST
      | 0b0 - Do nothing
      | 0b1 - Force TZ
  Action Port : ActionPort
  System Outputs2 : Subsystem  mask(System Outputs){ShowInLibBrowser=0}
      mask prompts: ShowInLibBrowser "Simulink:masks:CustCodeMaskParam1_MP"
      settings: CopyFcn=cccopyfcn(gcb)  OpenFcn=ccopenfcn('System Outputs Function')
      mask Help: eval('feval(''rtwprivate'',''rtwhelpview'',''rtw_sys_outputs_block'')');
      mask Display: disp('System\nOutputs');

== system npc_controller/CONTROL/STATE-MACHINE/CPU_CONTROL_100_A2_precharge_pfc_ok2/configGrid/FORCE_TZ/3P3W/System Outputs2 ==

== system npc_controller/CONTROL/STATE-MACHINE/CPU_CONTROL_100_A2_precharge_pfc_ok2/updateCalib/done/RESET_TZ/System Outputs2 ==

== system npc_controller/CONTROL/STATE-MACHINE/CPU_CONTROL_100_A2_precharge_pfc_ok2/updatePll3p/PLL/SRF_PLL/Integrator ==
  PI Out : Inport  OutDataTypeStr=single
  Accumulation : Subsystem  TreatAsAtomicUnit=on
  Add : Sum  AccumDataTypeStr=single
  Compare To Constant : simulink/Logic and Bit Operations/Compare To Constant  relop=>=  const=2*pi  OutDataTypeStr=boolean
  If : If  IfExpression=u1
  Merge : Merge
  Product : Product  OutDataTypeStr=single
  Reset Integrator : Subsystem  TreatAsAtomicUnit=on
  Ts : Constant  Value=Tsw  OutDataTypeStr=single
  Unit Delay : UnitDelay  SampleTime=-1  HasFrameUpgradeWarning=on
  wt : Outport
  wires:
  PI Out/1 -> Product/1
  Ts/1 -> Product/2
  Product/1 -> Add/1
  Add/1 -> Accumulation/1(In1), Compare To Constant/1
  Compare To Constant/1 -> If/1
  If/1 -> Reset Integrator/Action
  If/2 -> Accumulation/Action
  Reset Integrator/1(Out) -> Merge/1
  Accumulation/1(Out) -> Merge/2
  Merge/1 -> Unit Delay/1
  Unit Delay/1 -> wt/1, Add/2

== system npc_controller/CONTROL/STATE-MACHINE/CPU_CONTROL_100_A2_precharge_pfc_ok2/updatePll3p/PLL/SRF_PLL/PI ==
  Vq : Inport
  Ki : Gain  Gain=200
  Ki1 : Gain  Commented=on  Gain=200
  Kp : Gain  Gain=0.5
  Kp1 : Gain  Commented=on  Gain=0.5
  Sum : Sum  Inputs=|++
  Sum1 : Sum  Inputs=+|+
  Ts/2 : Gain  Gain=Tsw/2
  Unit Delay : UnitDelay  SampleTime=-1  HasFrameUpgradeWarning=on
  PI Out : Outport
  wires:
  Ts/2/1 -> Sum/1
  Sum1/1 -> PI Out/1
  Ki/1 -> Ts/2/1
  Vq/1 -> Ki/1, Kp/1  "Vq"
  Unit Delay/1 -> Sum/2
  Kp/1 -> Sum1/1
  Sum/1 -> Sum1/2, Unit Delay/1

== system npc_controller/CONTROL/STATE-MACHINE/CPU_CONTROL_100_A2_precharge_pfc_ok2/updatePll3p/PLL/SRF_PLL/Subsystem1 ==
  x[n] : Inport
  1 - Lambda : Gain  Gain=1 - 0.98
  Delay : Delay  DelayLength=1
  Gain{,1..7} (8 alike) : Gain  Commented=on  Gain=1/8
  Lambda : Gain  Gain=0.98
  Memory{,1..6} (7 alike) : Memory  Commented=on  InheritSampleTime=on
  Sum{,1..6} (7 alike) : Sum  Commented=on  Inputs=++|
  Sum7 : Sum  Inputs=|++
  y[n] : Outport
  wires:
  Sum7/1 -> y[n]/1, Delay/1
  Delay/1 -> Lambda/1
  1 - Lambda/1 -> Sum7/1
  x[n]/1 -> 1 - Lambda/1
  Lambda/1 -> Sum7/2
  Gain7/1 -> Sum6/1
  Sum5/1 -> Sum6/2
  Memory6/1 -> Gain7/1
  Memory5/1 -> Gain6/1, Memory6/1
  Sum4/1 -> Sum5/2
  Gain6/1 -> Sum5/1
  Gain5/1 -> Sum4/1
  Sum3/1 -> Sum4/2
  Memory4/1 -> Gain5/1, Memory5/1
  Memory3/1 -> Gain4/1, Memory4/1
  Sum2/1 -> Sum3/2
  Gain4/1 -> Sum3/1
  Gain3/1 -> Sum2/1
  Sum1/1 -> Sum2/2
  Gain2/1 -> Sum1/1
  Sum/1 -> Sum1/2
  Gain1/1 -> Sum/1
  Gain/1 -> Sum/2
  Memory2/1 -> Gain3/1, Memory3/1
  Memory1/1 -> Gain2/1, Memory2/1
  Memory/1 -> Gain1/1, Memory1/1

== system npc_controller/CONTROL/STATE-MACHINE/CPU_CONTROL_100_A2_precharge_pfc_ok2/updatePll3p/PLL/SRF_PLL/abc to dq ==
  note: wt
  note: wt
  note: wt
  a : Inport
  b : Inport  Port=2
  c : Inport  Port=3
  wt : Inport  Port=4
  (wt+120) : Sum  Inputs=|++
  (wt-120) : Sum  Inputs=|+-
  2pi_3 : Constant  Value=2*pi/3
  Add3 : Sum  Inputs=+++
  Cos3 : Trigonometry  Operator=cos
  Cos4 : Trigonometry  Operator=cos
  Cos5 : Trigonometry  Operator=cos
  Product5 : Product
  Product6 : Product
  Product7 : Product
  q1 : Gain  Gain=2/3
  q : Outport
  wires:
  [a] -> Product5/1
  Cos3/1 -> Product5/2
  wt/1 -> (wt+120)/1, (wt-120)/1, Cos3/1
  [ph] -> (wt+120)/2
  Product7/1 -> Add3/3
  a/1 -> [a]
  (wt+120)/1 -> Cos5/1
  Product6/1 -> Add3/2
  c/1 -> [c]
  [ph] -> (wt-120)/2
  (wt-120)/1 -> Cos4/1
  [b] -> Product6/1
  Cos4/1 -> Product6/2
  Product5/1 -> Add3/1
  Cos5/1 -> Product7/2
  b/1 -> [b]
  Add3/1 -> q1/1
  [c] -> Product7/1
  q1/1 -> q/1
  2pi_3/1 -> [ph]

== system npc_controller/CONTROL/STATE-MACHINE/CPU_CONTROL_100_A2_precharge_pfc_ok2/updatePll3p/PLL/Subsystem/Initialize at Zero Crossing ==
  In1 : Inport
  Trigger : TriggerPort  VariantControl=Variant
  OR : Logic  Operator=OR  IconShape=distinctive  AllPortsSameDT=off  OutDataTypeStr=boolean
  Unit Delay : UnitDelay  SampleTime=-1  HasFrameUpgradeWarning=on
  Out1 : Outport  InitialOutput=0  VectorParamsAs1DForOutWhenUnconnected=off
  wires:
  OR/1 -> Out1/1, Unit Delay/1
  Unit Delay/1 -> OR/2
  In1/1 -> OR/1

== system npc_controller/CONTROL/STATE-MACHINE/CPU_CONTROL_100_A2_precharge_pfc_ok2/updateSequencePhA/pol_final1/prot/System Outputs ==

== system npc_controller/CONTROL/STATE-MACHINE/CPU_CONTROL_100_A2_precharge_pfc_ok2/updateSequencePhA/pol_vxn1/neg/System Outputs1 ==

== system npc_controller/CONTROL/STATE-MACHINE/CPU_CONTROL_100_A2_precharge_pfc_ok2/updateSequencePhA/pol_vxn1/pos/System Outputs1 ==

== system npc_controller/CONTROL/STATE-MACHINE/CPU_CONTROL_100_A2_precharge_pfc_ok2/updateSequencePhA/pol_vxn1/zero/System Outputs1 ==

== system npc_controller/CONTROL/STATE-MACHINE/CPU_CONTROL_100_A2_precharge_pfc_ok2/updateSequencePhB/pol_final1/prot/System Outputs ==

== system npc_controller/CONTROL/STATE-MACHINE/CPU_CONTROL_100_A2_precharge_pfc_ok2/updateSequencePhB/pol_vxn1/neg/System Outputs1 ==

== system npc_controller/CONTROL/STATE-MACHINE/CPU_CONTROL_100_A2_precharge_pfc_ok2/updateSequencePhB/pol_vxn1/pos/System Outputs1 ==

== system npc_controller/CONTROL/STATE-MACHINE/CPU_CONTROL_100_A2_precharge_pfc_ok2/updateSequencePhB/pol_vxn1/zero/System Outputs1 ==

== system npc_controller/CONTROL/STATE-MACHINE/CPU_CONTROL_100_A2_precharge_pfc_ok2/updateSequencePhC/pol_final1/prot/System Outputs ==

== system npc_controller/CONTROL/STATE-MACHINE/CPU_CONTROL_100_A2_precharge_pfc_ok2/updateSequencePhC/pol_vxn1/neg/System Outputs1 ==

== system npc_controller/CONTROL/STATE-MACHINE/CPU_CONTROL_100_A2_precharge_pfc_ok2/updateSequencePhC/pol_vxn1/pos/System Outputs1 ==

== system npc_controller/CONTROL/STATE-MACHINE/CPU_CONTROL_100_A2_precharge_pfc_ok2/updateSequencePhC/pol_vxn1/zero/System Outputs1 ==

== system npc_controller/CONTROL/STATE-MACHINE/CPU_CONTROL_200_A2_precharge_pfc_ok2/configGrid/FORCE_TZ/1P/ALL_LEGS ==
  note: Note:
      | TZCCTL
      | 0b00 - High impedance
      | 0b01 - Force to HIGH
      | 0b10 - Force to LOW
      | 0b11 - Do nothing
      |
      | AQCSFRC
      | 0b00 - disables forced PWM
      | 0b01 - forces PWM to LOW
      | 0b10 - forces PWM to  HIGH
      |
      | TZFRC.bit.OST
      | 0b0 - Do nothing
      | 0b1 - Force TZ
  note: EALLOW;
      |
      | /*Force TZ*/
      | EPwm6Regs. TZFRC.bit.OST = 0b0; //do nothing
      | EPwm7Regs. TZFRC.bit.OST = 0b0;
      | EPwm8Regs. TZFRC.bit.OST = 0b0;
      | EPwm9Regs. TZFRC.bit.OST = 0b0;
      | EPwm10Regs. TZFRC.bit.OST = 0b0;
      | EPwm11Regs. TZFRC.bit.OST = 0b0;
      |
      | EDIS;
      |
      | //change ref for leg B and legC
  Action Port : ActionPort
  System Outputs2 : Subsystem  mask(System Outputs){ShowInLibBrowser=0}
      mask prompts: ShowInLibBrowser "Simulink:masks:CustCodeMaskParam1_MP"
      settings: CopyFcn=cccopyfcn(gcb)  OpenFcn=ccopenfcn('System Outputs Function')
      mask Help: eval('feval(''rtwprivate'',''rtwhelpview'',''rtw_sys_outputs_block'')');
      mask Display: disp('System\nOutputs');

== system npc_controller/CONTROL/STATE-MACHINE/CPU_CONTROL_200_A2_precharge_pfc_ok2/configGrid/FORCE_TZ/1P/LEG_A ==
  note: EALLOW;
      |
      | /*Force TZ*/
      | EPwm6Regs. TZFRC.bit.OST = 0b0; //do nothing
      | EPwm7Regs. TZFRC.bit.OST = 0b0;
      | EPwm8Regs. TZFRC.bit.OST = 0b1;
      | EPwm9Regs. TZFRC.bit.OST = 0b1;
      | EPwm10Regs. TZFRC.bit.OST = 0b1;
      | EPwm11Regs. TZFRC.bit.OST = 0b1;
      |
      | EDIS;
  note: Note:
      | TZCCTL
      | 0b00 - High impedance
      | 0b01 - Force to HIGH
      | 0b10 - Force to LOW
      | 0b11 - Do nothing
      |
      | AQCSFRC
      | 0b00 - disables forced PWM
      | 0b01 - forces PWM to LOW
      | 0b10 - forces PWM to  HIGH
      |
      | TZFRC.bit.OST
      | 0b0 - Do nothing
      | 0b1 - Force TZ
  Action Port : ActionPort
  System Outputs2 : Subsystem  mask(System Outputs){ShowInLibBrowser=0}
      mask prompts: ShowInLibBrowser "Simulink:masks:CustCodeMaskParam1_MP"
      settings: CopyFcn=cccopyfcn(gcb)  OpenFcn=ccopenfcn('System Outputs Function')
      mask Help: eval('feval(''rtwprivate'',''rtwhelpview'',''rtw_sys_outputs_block'')');
      mask Display: disp('System\nOutputs');

== system npc_controller/CONTROL/STATE-MACHINE/CPU_CONTROL_200_A2_precharge_pfc_ok2/configGrid/FORCE_TZ/1P/LEG_B ==
  note: Note:
      | TZCCTL
      | 0b00 - High impedance
      | 0b01 - Force to HIGH
      | 0b10 - Force to LOW
      | 0b11 - Do nothing
      |
      | AQCSFRC
      | 0b00 - disables forced PWM
      | 0b01 - forces PWM to LOW
      | 0b10 - forces PWM to  HIGH
      |
      | TZFRC.bit.OST
      | 0b0 - Do nothing
      | 0b1 - Force TZ
  note: EALLOW;
      |
      | /*Force TZ*/
      | EPwm6Regs. TZFRC.bit.OST = 0b1; //do nothing
      | EPwm7Regs. TZFRC.bit.OST = 0b1;
      | EPwm8Regs. TZFRC.bit.OST = 0b0;
      | EPwm9Regs. TZFRC.bit.OST = 0b0;
      | EPwm10Regs. TZFRC.bit.OST = 0b1;
      | EPwm11Regs. TZFRC.bit.OST = 0b1;
      |
      | EDIS;
  Action Port : ActionPort
  System Outputs2 : Subsystem  mask(System Outputs){ShowInLibBrowser=0}
      mask prompts: ShowInLibBrowser "Simulink:masks:CustCodeMaskParam1_MP"
      settings: CopyFcn=cccopyfcn(gcb)  OpenFcn=ccopenfcn('System Outputs Function')
      mask Help: eval('feval(''rtwprivate'',''rtwhelpview'',''rtw_sys_outputs_block'')');
      mask Display: disp('System\nOutputs');

== system npc_controller/CONTROL/STATE-MACHINE/CPU_CONTROL_200_A2_precharge_pfc_ok2/configGrid/FORCE_TZ/1P/LEG_C ==
  note: EALLOW;
      |
      | /*Force TZ*/
      | EPwm6Regs. TZFRC.bit.OST = 0b1; //do nothing
      | EPwm7Regs. TZFRC.bit.OST = 0b1;
      | EPwm8Regs. TZFRC.bit.OST = 0b1;
      | EPwm9Regs. TZFRC.bit.OST = 0b1;
      | EPwm10Regs. TZFRC.bit.OST = 0b0;
      | EPwm11Regs. TZFRC.bit.OST = 0b0;
      |
      | EDIS;
  note: Note:
      | TZCCTL
      | 0b00 - High impedance
      | 0b01 - Force to HIGH
      | 0b10 - Force to LOW
      | 0b11 - Do nothing
      |
      | AQCSFRC
      | 0b00 - disables forced PWM
      | 0b01 - forces PWM to LOW
      | 0b10 - forces PWM to  HIGH
      |
      | TZFRC.bit.OST
      | 0b0 - Do nothing
      | 0b1 - Force TZ
  Action Port : ActionPort
  System Outputs2 : Subsystem  mask(System Outputs){ShowInLibBrowser=0}
      mask prompts: ShowInLibBrowser "Simulink:masks:CustCodeMaskParam1_MP"
      settings: CopyFcn=cccopyfcn(gcb)  OpenFcn=ccopenfcn('System Outputs Function')
      mask Help: eval('feval(''rtwprivate'',''rtwhelpview'',''rtw_sys_outputs_block'')');
      mask Display: disp('System\nOutputs');

== system npc_controller/CONTROL/STATE-MACHINE/CPU_CONTROL_200_A2_precharge_pfc_ok2/configGrid/FORCE_TZ/3P3W/System Outputs2 ==

== system npc_controller/CONTROL/STATE-MACHINE/CPU_CONTROL_200_A2_precharge_pfc_ok2/updateCalib/done/RESET_TZ/System Outputs2 ==

== system npc_controller/CONTROL/STATE-MACHINE/CPU_CONTROL_200_A2_precharge_pfc_ok2/updatePll3p/PLL/SRF_PLL/Integrator ==
  PI Out : Inport  OutDataTypeStr=single
  Accumulation : Subsystem  TreatAsAtomicUnit=on
  Add : Sum  AccumDataTypeStr=single
  Compare To Constant : simulink/Logic and Bit Operations/Compare To Constant  relop=>=  const=2*pi  OutDataTypeStr=boolean
  If : If  IfExpression=u1
  Merge : Merge
  Product : Product  OutDataTypeStr=single
  Reset Integrator : Subsystem  TreatAsAtomicUnit=on
  Ts : Constant  Value=Tsw  OutDataTypeStr=single
  Unit Delay : UnitDelay  SampleTime=-1  HasFrameUpgradeWarning=on
  wt : Outport
  wires:
  PI Out/1 -> Product/1
  Ts/1 -> Product/2
  Product/1 -> Add/1
  Add/1 -> Accumulation/1(In1), Compare To Constant/1
  Compare To Constant/1 -> If/1
  If/1 -> Reset Integrator/Action
  If/2 -> Accumulation/Action
  Reset Integrator/1(Out) -> Merge/1
  Accumulation/1(Out) -> Merge/2
  Merge/1 -> Unit Delay/1
  Unit Delay/1 -> wt/1, Add/2

== system npc_controller/CONTROL/STATE-MACHINE/CPU_CONTROL_200_A2_precharge_pfc_ok2/updatePll3p/PLL/SRF_PLL/PI ==
  Vq : Inport
  Ki : Gain  Gain=200
  Ki1 : Gain  Commented=on  Gain=200
  Kp : Gain  Gain=0.5
  Kp1 : Gain  Commented=on  Gain=0.5
  Sum : Sum  Inputs=|++
  Sum1 : Sum  Inputs=+|+
  Ts/2 : Gain  Gain=Tsw/2
  Unit Delay : UnitDelay  SampleTime=-1  HasFrameUpgradeWarning=on
  PI Out : Outport
  wires:
  Ts/2/1 -> Sum/1
  Sum1/1 -> PI Out/1
  Ki/1 -> Ts/2/1
  Vq/1 -> Ki/1, Kp/1  "Vq"
  Unit Delay/1 -> Sum/2
  Kp/1 -> Sum1/1
  Sum/1 -> Sum1/2, Unit Delay/1
